simulink model "Control_system"  (R2022b)
settings: Solver=VariableStepAuto  StartTime=0  StopTime=Tend  FixedStep=0.01  MaxStep=0.1  RelTol=1  AbsTol=1
values from neighbouring files (symbols this model uses):
  D_Upper_Limit = 0    [Insulin_controller.m]
  G = Gp/Paz.Vg    [G_I_Model.m]    (also in Insulin_controller.m = Gmis)
  Gref = Gref+1    [Insulin_controller.m]
  I_conversione = Paz.I_conversione    [Glucose_insuline_response.m]    (also in Insulin_controller.m; patient_generator.m = conc_insulina_litro_plasma_Kg)
  kernel = ones(1,windowWidth) / windowWidth    [Insulin_controller.m]
  Pasti = [0,0,0]    [Glucose_insuline_response.m]    (also in Insulin_controller.m = Pasti0+0.2*(-1+2*rand(3,1)).*Pasti0; patient_generator.m = Pasti0)
  Tend = Paz.Tend    [Glucose_insuline_response.m]    (also in Insulin_controller.m; patient_generator.m = 1440)
  Tpasti = Tpasti0    [Glucose_insuline_response.m]    (also in Insulin_controller.m = Tpasti0+delta_T)
  x0 = y(end,1:13)'    [Glucose_insuline_response.m]    (also in Insulin_controller.m; patient_generator.m = [Gp Gt Il Ip I1 Id Qsto1 Qsto2 Qgut X Isc1 Isc2 Dstato])
undefined symbols (not defined in the file or in its folder): Af, Bf, Cf, Df, Paz
libraries: simulink x1
settings Model: Creator=federico  LastModifiedBy=federico
settings SolverCC: MaxConsecutiveMinStep=auto
settings DataIOCC: SaveFormat=Array  SignalLoggingSaveFormat=ModelDataLogs  ReturnWorkspaceOutputs=off
settings OptimizationCC: BlockReduction=off  BooleanDataType=off  InitFltsAndDblsToZero=on  LifeSpan=inf
settings DebuggingCC: SaveWithParameterizedLinksMsg=none  UnderspecifiedInitializationDetection=Classic  MergeDetectMultiDrivingBlocksExec=none  SignalResolutionControl=TryResolveAllWithWarning  MultiTaskDSMMsg=warning  MultiTaskCondExecSysMsg=none  UnconnectedInputMsg=warning  UnconnectedOutputMsg=warning  UnconnectedLineMsg=warning  SFUnexpectedBacktrackingDiag=warning  SFNoUnconditionalDefaultTransitionDiag=warning  SFExecutionAtInitializationDiag=none  SFMachineParentedDataDiag=warning  ArithmeticOperatorsInVariantConditions=warning
settings HardwareCC: ProdBitPerPointer=32  ProdBitPerSizeT=32  ProdBitPerPtrDiffT=32  ProdLargestAtomicFloat=None  ProdIntDivRoundTo=Undefined  ProdEndianess=Unspecified  ProdWordSize=32  ProdHWDeviceType=32-bit Generic  TargetUnknown=on
settings ModelReferenceCC: PropagateSignalLabelsOutOfModel=off
settings CodeAppCC: StateflowObjectComments=on
settings GRTTargetCC: TargetFcnLib=ansi_tfl_tmw.mat  TargetLangStandard=C89/C90 (ANSI)  CombineOutputUpdateFcns=off  GRTInterface=on
settings ConfigComp: CovMetricSettings=dw  CovSaveCumulativeToWorkspaceVar=on  CovSaveSingleToWorkspaceVar=on

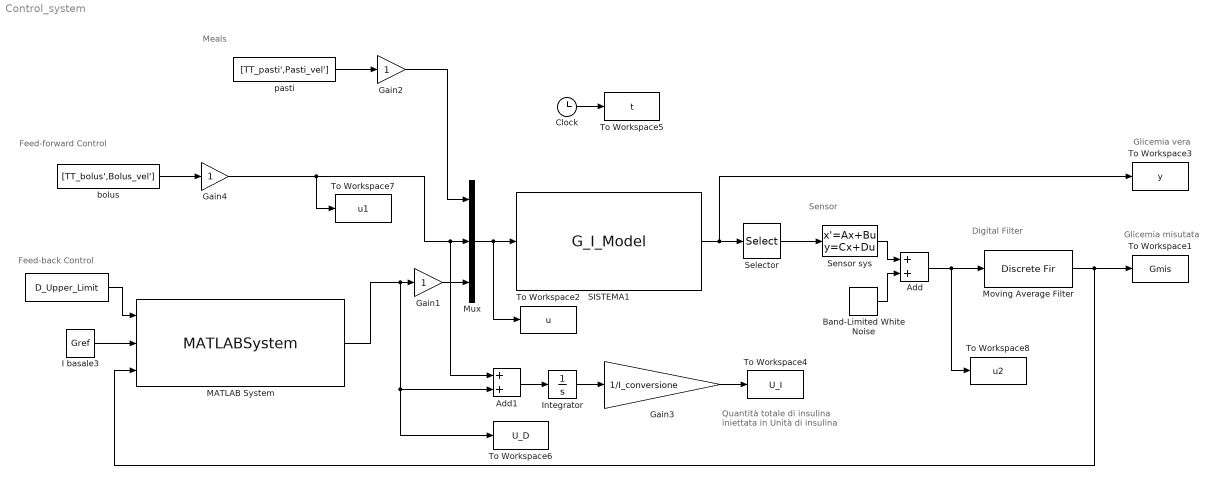
== system Control_system ==
  note: Quantità totale di insulina
      | iniettata in Unità di insulina
  note: Glicemia misutata
  note: Glicemia vera
  note: Digital Filter
  note: Sensor
  note: Meals
  note: Feed-forward Control
  note: Feed-back Control
  " " : Constant  Value=D_Upper_Limit
  Add : Sum
  Add1 : Sum
  Band-Limited White Noise : simulink/Sources/Band-Limited White Noise  Cov=[10]  Ts=1  seed=[23341]
  Clock : Clock
  Gain1 : Gain
  Gain2 : Gain
  Gain3 : Gain  Gain=1/I_conversione
  Gain4 : Gain
  I basale3 : Constant  Value=Gref
  Integrator : Integrator
  MATLAB System : MATLABSystem  System=Derivative_module  SimulateUsing=Code generation
      mask Type: Derivative_module
      mask Display:
      | disp('Derivative_module');
      | port_label('input',1,'D_UPPER_LIMIT');
      | port_label('input',2,'Gref');
      | port_label('input',3,'u');
      | port_label('output',1,'y');
  Moving Average Filter : DiscreteFir  FilterStructure=Direct form symmetric  Coefficients=kernel  InitialStates=G(Tend)
  Mux : Mux  Inputs=3
  SISTEMA1 : S-Function  FunctionName=G_I_Model  Parameters=Tpasti,Pasti,Paz,x0  SFunctionDeploymentMode=off  EnableBusSupport=off
  Selector : Selector  InputPortWidth=19  IndexOptions=Index vector (dialog)  Indices=[14]  OutputSizes=1
  Sensor sys : StateSpace  A=Af  B=Bf  C=Cf  D=Df  InitialCondition=G(Tend)/Cf
  To Workspace1 : ToWorkspace  VariableName=Gmis  SampleTime=1
  To Workspace2 : ToWorkspace  VariableName=u  SampleTime=1
  To Workspace3 : ToWorkspace  VariableName=y  SampleTime=1
  To Workspace4 : ToWorkspace  VariableName=U_I  SampleTime=1
  To Workspace5 : ToWorkspace  VariableName=t  SampleTime=1
  To Workspace6 : ToWorkspace  VariableName=U_D  SampleTime=1
  To Workspace7 : ToWorkspace  VariableName=u1  SampleTime=1
  To Workspace8 : ToWorkspace  VariableName=u2  SampleTime=1
  bolus : FromWorkspace  VariableName=[TT_bolus',Bolus_vel']  ZeroCross=off
  pasti : FromWorkspace  VariableName=[TT_pasti',Pasti_vel']  ZeroCross=off
  wires:
  Clock/1 -> To Workspace5/1
  SISTEMA1/1 -> Selector/1, To Workspace3/1
  Mux/1 -> To Workspace2/1, SISTEMA1/1
  Selector/1 -> Sensor sys/1
  Sensor sys/1 -> Add/1
  pasti/1 -> Gain2/1
  bolus/1 -> Gain4/1
  Integrator/1 -> Gain3/1
  Gain3/1 -> To Workspace4/1
  Band-Limited White Noise/1 -> Add/2
  Add/1 -> Moving Average Filter/1, To Workspace8/1
  Moving Average Filter/1 -> MATLAB System/3, To Workspace1/1
  I basale3/1 -> MATLAB System/2
  Add1/1 -> Integrator/1
  " "/1 -> MATLAB System/1
  Gain2/1 -> Mux/1
  Gain4/1 -> To Workspace7/1, Mux/2, Add1/1
  MATLAB System/1 -> Add1/2, To Workspace6/1, Gain1/1
  Gain1/1 -> Mux/3
